simulink library "simetranss"  (R2024b)
settings: Solver=VariableStepAuto  StartTime=0.0  StopTime=10.0  RelTol=1e-3
PostLoadFcn:
  | Ts=1e-6
InitFcn:
  | Ts=1e-6
undefined symbols (not defined in the file): C, C_601, C_603, C_606, CC, Csnu, Csnubber, DiscIntNeverNeededParam, DPL, DPL1ph, FluxTable, ft2km, gcbh, h, Half, Imap2, L, L_601, L_603, L_606, Lbase, LpejoSw, Newton, R_601, R_603, R_606, Raphson, ResistanceM, Roff, Ron, RotorAngles, Rsnu, Rsnubber, Rt4, SampleTime, simetran, sps, sps_rtmsupport, StatorCurrents, T_2wind_ratio, T_Lpu, T_Lpu_pri, T_Rpu, T_Rpu_pri, T_Vpri, T_Vpri_15comp, T_Vsec, Ti, Ts_Power, Z, Zbase, Zm
libraries: fl_lib x248, ee_lib x146, nesl_utility x122, $bdroot x29, simulink x15, eeGeneralControl x2, spsStairGeneratorLib x2, artemis x1
(part 4 of 12)

== system simetranss/FPGA/MATE 2-level inverter backup ==
  gate : Inport
  Demux2 : Demux  Outputs=2
  Pejovic L/C switch2 : Subsystem  mask(Pejovic Switch){Lon=Lon, Ts=Ts}
      mask prompts: Lon "Selected equivalent ON inductance (H)"; Ts "Sample Time (s)"
      mask help:
      | Pevovic switch model in SimScape
      |
      | In the Pejovic model, Ts/Lon=Coff/Ts (Backward Euler)
      |
      |
      | Implements a single phase switch model using the Pejovic constant admittance method.
      | The user only has to select the equivalent ON-state inductance of the model, the corresponding Capacitance is computed internally.
      |
      | Input signals;
      |
      | sw: the switch gate value (1 for ON , 0 for OFF)
      mask init:
      | Coff=Ts*Ts/Lon;
      | Rsw=Lon/Ts;
      | 
      | if Ts>2e-6
      |     warndlg(['Sample Time of ' num2str(Ts) ' s. may be somehow large for the Pejovic switch to be accurate. Sample time below 2 us are recommended.'])
      | end
      mask Display: disp(['Pswitch'])
  Pejovic L/C switch3 : Subsystem  mask(Pejovic Switch){Lon=Lon, Ts=Ts}
      mask prompts: Lon "Selected equivalent ON inductance (H)"; Ts "Sample Time (s)"
      mask help:
      | Pevovic switch model in SimScape
      |
      | In the Pejovic model, Ts/Lon=Coff/Ts (Backward Euler)
      |
      |
      | Implements a single phase switch model using the Pejovic constant admittance method.
      | The user only has to select the equivalent ON-state inductance of the model, the corresponding Capacitance is computed internally.
      |
      | Input signals;
      |
      | sw: the switch gate value (1 for ON , 0 for OFF)
      mask init:
      | Coff=Ts*Ts/Lon;
      | Rsw=Lon/Ts;
      | 
      | if Ts>2e-6
      |     warndlg(['Sample Time of ' num2str(Ts) ' s. may be somehow large for the Pejovic switch to be accurate. Sample time below 2 us are recommended.'])
      | end
      mask Display: disp(['Pswitch'])
  V+ : PMIOPort  Side=Left
  Vout : PMIOPort  Port=2  Side=Right
  V- : PMIOPort  Port=3  Side=Left
  wires:
  Pejovic L/C switch3/2(Xout) -> Pejovic L/C switch2/2(Xin)
  Pejovic L/C switch2/2(Xout) -> Pejovic L/C switch3/2(Xin)
  gate/1 -> Demux2/1
  Demux2/1 -> Pejovic L/C switch2/1(gate)
  Demux2/2 -> Pejovic L/C switch3/1(gate)
  connections:
  Pejovic L/C switch3/RConn1 -- V-/RConn1
  V+/RConn1 -- Pejovic L/C switch2/LConn1
  Pejovic L/C switch3/LConn1 -- Pejovic L/C switch2/RConn1 -- Vout/RConn1

== system simetranss/FPGA/MATE 2level_Inverter SwitchingFunction(2ph) ==
  g : Inport
  Add : Sum  Inputs=+
  Controlled Current Source1 : fl_lib/Electrical/Electrical Sources/Controlled Current Source
  Controlled Voltage Source : fl_lib/Electrical/Electrical Sources/Controlled Voltage Source
  Controlled Voltage Source1 : fl_lib/Electrical/Electrical Sources/Controlled Voltage Source
  Current Sensor : fl_lib/Electrical/Electrical Sensors/Current Sensor
  Current Sensor1 : fl_lib/Electrical/Electrical Sensors/Current Sensor
  Demux : Demux  Outputs=2
  Mux : Mux  Inputs=2
  PS-Simulink Converter : nesl_utility/PS-Simulink Converter  PhysicalDomain=network_engine_domain  SubClassName=ps_output  LeftPortType=input  RightPortType=output  PseudoPeriodic=off  Frequencies=[]  VectorFormat=inherit  Unit=inherit  AffineConversion=off
  PS-Simulink Converter1 : nesl_utility/PS-Simulink Converter  PhysicalDomain=network_engine_domain  SubClassName=ps_output  LeftPortType=input  RightPortType=output  PseudoPeriodic=off  Frequencies=[]  VectorFormat=inherit  Unit=inherit  AffineConversion=off
  PS-Simulink Converter3 : nesl_utility/PS-Simulink Converter  PhysicalDomain=network_engine_domain  SubClassName=ps_output  LeftPortType=input  RightPortType=output  PseudoPeriodic=off  Frequencies=[]  VectorFormat=inherit  Unit=inherit  AffineConversion=off
  Resistor : fl_lib/Electrical/Electrical Elements/Resistor  R=Ron Ohm  i_specify=off  i_priority=None  i=0 A  i_nominal_specify=off  i_nominal_value=1  i_nominal_unit=A  v_specify=off  v_priority=None  v=0 V  v_nominal_specify=off  v_nominal_value=1  v_nominal_unit=V
  Resistor1 : fl_lib/Electrical/Electrical Elements/Resistor  R=Ron Ohm  i_specify=off  i_priority=None  i=0 A  i_nominal_specify=off  i_nominal_value=1  i_nominal_unit=A  v_specify=off  v_priority=None  v=0 V  v_nominal_specify=off  v_nominal_value=1  v_nominal_unit=V
  SW : $bdroot/FPGA/MATE 2level_Inverter  SwitchingFunction(3ph)/SW  SystemSampleTime=-1  VariantActivationTime=update diagram  AllowFlexibleInterface=on  Latency=0  AutoFrameSizeCalculation=off
  Selector : Selector  InputPortWidth=4  IndexOptions=Index vector (dialog)  Indices=[1 3]  OutputSizes=1
  Selector1 : Selector  InputPortWidth=4  IndexOptions=Index vector (dialog)  Indices=[2 4]  OutputSizes=1
  Simulink-PS Converter : nesl_utility/Simulink-PS Converter  PhysicalDomain=network_engine_domain  SubClassName=ps_input  LeftPortType=input  RightPortType=output  PseudoPeriodic=off  Frequencies=[]  NoiseDistribution=none  NoiseParameters=[]  Unit=1  AffineConversion=off  FilteringAndDerivatives=provide  SimscapeFilterOrder=1  InputFilterTimeConstant=0.001  UdotUserProvided=0
  Simulink-PS Converter1 : nesl_utility/Simulink-PS Converter  PhysicalDomain=network_engine_domain  SubClassName=ps_input  LeftPortType=input  RightPortType=output  PseudoPeriodic=off  Frequencies=[]  NoiseDistribution=none  NoiseParameters=[]  Unit=1  AffineConversion=off  FilteringAndDerivatives=provide  SimscapeFilterOrder=1  InputFilterTimeConstant=0.001  UdotUserProvided=0
  Simulink-PS Converter2 : nesl_utility/Simulink-PS Converter  PhysicalDomain=network_engine_domain  SubClassName=ps_input  LeftPortType=input  RightPortType=output  PseudoPeriodic=off  Frequencies=[]  NoiseDistribution=none  NoiseParameters=[]  Unit=1  AffineConversion=off  FilteringAndDerivatives=provide  SimscapeFilterOrder=1  InputFilterTimeConstant=0.001  UdotUserProvided=0
  Unit Delay : UnitDelay  SampleTime=Ts  HasFrameUpgradeWarning=on
  Unit Delay1 : UnitDelay  SampleTime=Ts  HasFrameUpgradeWarning=on
  Voltage Sensor : fl_lib/Electrical/Electrical Sensors/Voltage Sensor
  V+ : PMIOPort  Side=Right
  V- : PMIOPort  Port=2  Side=Right
  + : PMIOPort  Port=3  Side=Left
  - : PMIOPort  Port=4  Side=Left
  wires:
  Add/1 -> Simulink-PS Converter/1
  g/1 -> Selector1/1, Selector/1
  SW/2 -> Unit Delay1/1
  SW/1 -> Unit Delay/1
  Unit Delay/1 -> Add/1
  PS-Simulink Converter1/1 -> SW/3
  PS-Simulink Converter/1 -> Mux/1
  PS-Simulink Converter3/1 -> Mux/2
  Mux/1 -> SW/4
  Demux/2 -> Simulink-PS Converter2/1
  Demux/1 -> Simulink-PS Converter1/1
  Unit Delay1/1 -> Demux/1
  Selector/1 -> SW/1
  Selector1/1 -> SW/2
  connections:
  Current Sensor/RConn2 -- Resistor/LConn1
  Controlled Voltage Source/LConn1 -- Current Sensor/LConn1
  Simulink-PS Converter/RConn1 -- Controlled Current Source1/RConn1
  PS-Simulink Converter/LConn1 -- Current Sensor/RConn1
  Simulink-PS Converter1/RConn1 -- Controlled Voltage Source/RConn1
  Controlled Voltage Source/RConn2 -- Controlled Current Source1/LConn1 -- Voltage Sensor/RConn2 -- V-/RConn1 -- Controlled Voltage Source1/RConn2
  Controlled Current Source1/RConn2 -- Voltage Sensor/LConn1 -- V+/RConn1
  PS-Simulink Converter1/LConn1 -- Voltage Sensor/RConn1
  Current Sensor1/RConn2 -- Resistor1/LConn1
  +/RConn1 -- Resistor/RConn1
  -/RConn1 -- Resistor1/RConn1
  PS-Simulink Converter3/LConn1 -- Current Sensor1/RConn1
  Current Sensor1/LConn1 -- Controlled Voltage Source1/LConn1
  Simulink-PS Converter2/RConn1 -- Controlled Voltage Source1/RConn1

== system simetranss/FPGA/MATE 2level_Inverter SwitchingFunction(3ph) ==
  g : Inport
  Add : Sum  Inputs=+
  Controlled Current Source1 : fl_lib/Electrical/Electrical Sources/Controlled Current Source
  Controlled Voltage Source : fl_lib/Electrical/Electrical Sources/Controlled Voltage Source
  Controlled Voltage Source1 : fl_lib/Electrical/Electrical Sources/Controlled Voltage Source
  Controlled Voltage Source2 : fl_lib/Electrical/Electrical Sources/Controlled Voltage Source
  Current Sensor : fl_lib/Electrical/Electrical Sensors/Current Sensor
  Current Sensor1 : fl_lib/Electrical/Electrical Sensors/Current Sensor
  Current Sensor2 : fl_lib/Electrical/Electrical Sensors/Current Sensor
  Demux : Demux  Outputs=3
  Mux : Mux  Inputs=3
  PS-Simulink Converter{,1..3} (4 alike) : nesl_utility/PS-Simulink Converter  PhysicalDomain=network_engine_domain  SubClassName=ps_output  LeftPortType=input  RightPortType=output  PseudoPeriodic=off  Frequencies=[]  VectorFormat=inherit  Unit=inherit  AffineConversion=off
  Phase Splitter : ee_lib/Connectors & References/Phase Splitter
  Resistor : fl_lib/Electrical/Electrical Elements/Resistor  R=Ron Ohm  i_specify=off  i_priority=None  i=0 A  i_nominal_specify=off  i_nominal_value=1  i_nominal_unit=A  v_specify=off  v_priority=None  v=0 V  v_nominal_specify=off  v_nominal_value=1  v_nominal_unit=V
  Resistor1 : fl_lib/Electrical/Electrical Elements/Resistor  R=Ron Ohm  i_specify=off  i_priority=None  i=0 A  i_nominal_specify=off  i_nominal_value=1  i_nominal_unit=A  v_specify=off  v_priority=None  v=0 V  v_nominal_specify=off  v_nominal_value=1  v_nominal_unit=V
  Resistor2 : fl_lib/Electrical/Electrical Elements/Resistor  R=Ron Ohm  i_specify=off  i_priority=None  i=0 A  i_nominal_specify=off  i_nominal_value=1  i_nominal_unit=A  v_specify=off  v_priority=None  v=0 V  v_nominal_specify=off  v_nominal_value=1  v_nominal_unit=V
  SW : Subsystem
  Selector : Selector  InputPortWidth=6  IndexOptions=Index vector (dialog)  Indices=[1 3 5]  OutputSizes=1
  Selector1 : Selector  InputPortWidth=6  IndexOptions=Index vector (dialog)  Indices=[1 3 5]+1  OutputSizes=1
  Simulink-PS Converter{,1..3} (4 alike) : nesl_utility/Simulink-PS Converter  PhysicalDomain=network_engine_domain  SubClassName=ps_input  LeftPortType=input  RightPortType=output  PseudoPeriodic=off  Frequencies=[]  NoiseDistribution=none  NoiseParameters=[]  Unit=1  AffineConversion=off  FilteringAndDerivatives=provide  SimscapeFilterOrder=1  InputFilterTimeConstant=0.001  UdotUserProvided=0
  Unit Delay : UnitDelay  SampleTime=Ts  HasFrameUpgradeWarning=on
  Unit Delay1 : UnitDelay  SampleTime=Ts  HasFrameUpgradeWarning=on
  Voltage Sensor : fl_lib/Electrical/Electrical Sensors/Voltage Sensor
  abc : PMIOPort  Side=Left
  V+ : PMIOPort  Port=2  Side=Right
  V- : PMIOPort  Port=3  Side=Right
  wires:
  Selector1/1 -> SW/2(gl)
  Selector/1 -> SW/1(gu)
  Unit Delay1/1 -> Demux/1
  Demux/1 -> Simulink-PS Converter1/1
  Demux/2 -> Simulink-PS Converter2/1
  Demux/3 -> Simulink-PS Converter3/1
  Mux/1 -> SW/4(Iac)
  PS-Simulink Converter2/1 -> Mux/3
  PS-Simulink Converter3/1 -> Mux/2
  PS-Simulink Converter/1 -> Mux/1
  PS-Simulink Converter1/1 -> SW/3(Vdc)
  Unit Delay/1 -> Add/1
  SW/1(Idc) -> Unit Delay/1
  SW/2(Vac) -> Unit Delay1/1
  g/1 -> Selector/1, Selector1/1
  Add/1 -> Simulink-PS Converter/1
  connections:
  Controlled Voltage Source2/LConn1 -- Current Sensor2/LConn1
  Simulink-PS Converter3/RConn1 -- Controlled Voltage Source2/RConn1
  Simulink-PS Converter2/RConn1 -- Controlled Voltage Source1/RConn1
  Current Sensor1/LConn1 -- Controlled Voltage Source1/LConn1
  PS-Simulink Converter2/LConn1 -- Current Sensor2/RConn1
  PS-Simulink Converter3/LConn1 -- Current Sensor1/RConn1
  Resistor2/RConn1 -- Phase Splitter/RConn3
  Resistor1/RConn1 -- Phase Splitter/RConn2
  Resistor/RConn1 -- Phase Splitter/RConn1
  Phase Splitter/LConn1 -- abc/RConn1
  Current Sensor2/RConn2 -- Resistor2/LConn1
  Current Sensor1/RConn2 -- Resistor1/LConn1
  PS-Simulink Converter1/LConn1 -- Voltage Sensor/RConn1
  V+/RConn1 -- Voltage Sensor/LConn1 -- Controlled Current Source1/RConn2
  Controlled Voltage Source2/RConn2 -- Controlled Voltage Source1/RConn2 -- V-/RConn1 -- Voltage Sensor/RConn2 -- Controlled Current Source1/LConn1 -- Controlled Voltage Source/RConn2
  Simulink-PS Converter1/RConn1 -- Controlled Voltage Source/RConn1
  PS-Simulink Converter/LConn1 -- Current Sensor/RConn1
  Simulink-PS Converter/RConn1 -- Controlled Current Source1/RConn1
  Controlled Voltage Source/LConn1 -- Current Sensor/LConn1
  Current Sensor/RConn2 -- Resistor/LConn1

== system simetranss/FPGA/MATE 2level_InverterSWHIZ ==
  g : Inport
  CCS : fl_lib/Electrical/Electrical Sources/Controlled Current Source
  CVS : fl_lib/Electrical/Electrical Sources/Controlled Voltage Source
  Constant : Constant  Value=[Gpp Ts/Gip min_charge]
  Isensor : fl_lib/Electrical/Electrical Sensors/Current Sensor
  PS-Simulink Converter : nesl_utility/PS-Simulink Converter  PhysicalDomain=network_engine_domain  SubClassName=ps_output  LeftPortType=input  RightPortType=output  PseudoPeriodic=off  Frequencies=[]  VectorFormat=inherit  Unit=inherit  AffineConversion=off
  PS-Simulink Converter1 : nesl_utility/PS-Simulink Converter  PhysicalDomain=network_engine_domain  SubClassName=ps_output  LeftPortType=input  RightPortType=output  PseudoPeriodic=off  Frequencies=[]  VectorFormat=inherit  Unit=inherit  AffineConversion=off
  R : fl_lib/Electrical/Electrical Elements/Resistor  R=Ron Ohm  i_specify=off  i_priority=None  i=0 A  i_nominal_specify=off  i_nominal_value=1  i_nominal_unit=A  v_specify=off  v_priority=None  v=0 V  v_nominal_specify=off  v_nominal_value=1  v_nominal_unit=V
  SW : Subsystem
  Selector : Selector  InputPortWidth=2  IndexOptions=Index vector (dialog)  Indices=[1 ]  OutputSizes=1
  Selector1 : Selector  InputPortWidth=2  IndexOptions=Index vector (dialog)  Indices=[2 ]  OutputSizes=1
  Simulink-PS Converter : nesl_utility/Simulink-PS Converter  PhysicalDomain=network_engine_domain  SubClassName=ps_input  LeftPortType=input  RightPortType=output  PseudoPeriodic=off  Frequencies=[]  NoiseDistribution=none  NoiseParameters=[]  Unit=1  AffineConversion=off  FilteringAndDerivatives=provide  SimscapeFilterOrder=1  InputFilterTimeConstant=0.001  UdotUserProvided=0
  Simulink-PS Converter1 : nesl_utility/Simulink-PS Converter  PhysicalDomain=network_engine_domain  SubClassName=ps_input  LeftPortType=input  RightPortType=output  PseudoPeriodic=off  Frequencies=[]  NoiseDistribution=none  NoiseParameters=[]  Unit=1  AffineConversion=off  FilteringAndDerivatives=provide  SimscapeFilterOrder=1  InputFilterTimeConstant=0.001  UdotUserProvided=0
  Unit Delay2 : UnitDelay  SampleTime=Ts  HasFrameUpgradeWarning=on
  Unit Delay3 : UnitDelay  SampleTime=Ts  HasFrameUpgradeWarning=on
  Vsensor : fl_lib/Electrical/Electrical Sensors/Voltage Sensor
  V+ : PMIOPort  Side=Left
  V- : PMIOPort  Port=2  Side=Left
  A : PMIOPort  Port=3  Side=Right
  wires:
  Constant/1 -> SW/5(params)
  Unit Delay3/1 -> SW/3(Vdc)
  Unit Delay2/1 -> SW/4(Iac)
  SW/2(Vac) -> Simulink-PS Converter1/1
  SW/1(Idc) -> Simulink-PS Converter/1
  g/1 -> Selector/1, Selector1/1
  PS-Simulink Converter1/1 -> Unit Delay3/1
  PS-Simulink Converter/1 -> Unit Delay2/1
  Selector/1 -> SW/1(gu)
  Selector1/1 -> SW/2(gl)
  connections:
  Isensor/RConn2 -- CVS/LConn1
  R/LConn1 -- Isensor/LConn1
  Simulink-PS Converter/RConn1 -- CCS/RConn1
  PS-Simulink Converter/LConn1 -- Isensor/RConn1
  Simulink-PS Converter1/RConn1 -- CVS/RConn1
  CCS/LConn1 -- Vsensor/RConn2 -- V-/RConn1 -- CVS/RConn2
  CCS/RConn2 -- Vsensor/LConn1 -- V+/RConn1
  PS-Simulink Converter1/LConn1 -- Vsensor/RConn1
  A/RConn1 -- R/RConn1

== system simetranss/FPGA/MATE 3levelNPC_Inverter SwitchingFunction(3ph) ==
  g : Inport
  Add : Sum  Inputs=+
  Add1 : Sum  Inputs=+
  Controlled Current Source1 : fl_lib/Electrical/Electrical Sources/Controlled Current Source
  Controlled Current Source2 : fl_lib/Electrical/Electrical Sources/Controlled Current Source
  Controlled Voltage Source : fl_lib/Electrical/Electrical Sources/Controlled Voltage Source
  Controlled Voltage Source1 : fl_lib/Electrical/Electrical Sources/Controlled Voltage Source
  Controlled Voltage Source2 : fl_lib/Electrical/Electrical Sources/Controlled Voltage Source
  Current Sensor : fl_lib/Electrical/Electrical Sensors/Current Sensor
  Current Sensor1 : fl_lib/Electrical/Electrical Sensors/Current Sensor
  Current Sensor2 : fl_lib/Electrical/Electrical Sensors/Current Sensor
  Demux : Demux  Outputs=3
  Mux : Mux  Inputs=3
  PS-Simulink Converter{,1..4} (5 alike) : nesl_utility/PS-Simulink Converter  PhysicalDomain=network_engine_domain  SubClassName=ps_output  LeftPortType=input  RightPortType=output  PseudoPeriodic=off  Frequencies=[]  VectorFormat=inherit  Unit=inherit  AffineConversion=off
  Phase Splitter : ee_lib/Connectors & References/Phase Splitter
  Q1 : Selector  InputPortWidth=12  IndexOptions=Index vector (dialog)  Indices=[1 5 9]  OutputSizes=[(-2)]
  Q2 : Selector  InputPortWidth=12  IndexOptions=Index vector (dialog)  Indices=[1 5 9]+1  OutputSizes=[(-2)]
  Q3 : Selector  InputPortWidth=12  IndexOptions=Index vector (dialog)  Indices=[1 5 9]+2  OutputSizes=[(-2)]
  Q4 : Selector  InputPortWidth=12  IndexOptions=Index vector (dialog)  Indices=[1 5 9]+3  OutputSizes=[(-2)]
  Resistor : fl_lib/Electrical/Electrical Elements/Resistor  R=2*Ron Ohm  i_specify=off  i_priority=None  i=0 A  i_nominal_specify=off  i_nominal_value=1  i_nominal_unit=A  v_specify=off  v_priority=None  v=0 V  v_nominal_specify=off  v_nominal_value=1  v_nominal_unit=V
  Resistor1 : fl_lib/Electrical/Electrical Elements/Resistor  R=2*Ron Ohm  i_specify=off  i_priority=None  i=0 A  i_nominal_specify=off  i_nominal_value=1  i_nominal_unit=A  v_specify=off  v_priority=None  v=0 V  v_nominal_specify=off  v_nominal_value=1  v_nominal_unit=V
  Resistor2 : fl_lib/Electrical/Electrical Elements/Resistor  R=2*Ron Ohm  i_specify=off  i_priority=None  i=0 A  i_nominal_specify=off  i_nominal_value=1  i_nominal_unit=A  v_specify=off  v_priority=None  v=0 V  v_nominal_specify=off  v_nominal_value=1  v_nominal_unit=V
  SW : Subsystem
  Simulink-PS Converter{,1..4} (5 alike) : nesl_utility/Simulink-PS Converter  PhysicalDomain=network_engine_domain  SubClassName=ps_input  LeftPortType=input  RightPortType=output  PseudoPeriodic=off  Frequencies=[]  NoiseDistribution=none  NoiseParameters=[]  Unit=1  AffineConversion=off  FilteringAndDerivatives=provide  SimscapeFilterOrder=1  InputFilterTimeConstant=0.001  UdotUserProvided=0
  Unit Delay : UnitDelay  SampleTime=Ts  HasFrameUpgradeWarning=on
  Unit Delay1 : UnitDelay  SampleTime=Ts  HasFrameUpgradeWarning=on
  Unit Delay2 : UnitDelay  SampleTime=Ts  HasFrameUpgradeWarning=on
  Voltage Sensor : fl_lib/Electrical/Electrical Sensors/Voltage Sensor
  Voltage Sensor1 : fl_lib/Electrical/Electrical Sensors/Voltage Sensor
  abc : PMIOPort  Side=Right
  V+ : PMIOPort  Port=2  Side=Left
  Vn : PMIOPort  Port=3  Side=Left
  V- : PMIOPort  Port=4  Side=Left
  wires:
  Q4/1 -> SW/4(g4)
  Q3/1 -> SW/3(g3)
  Q2/1 -> SW/2(g2)
  Q1/1 -> SW/1(g1)
  Unit Delay1/1 -> Demux/1
  Demux/1 -> Simulink-PS Converter1/1
  Demux/2 -> Simulink-PS Converter2/1
  Demux/3 -> Simulink-PS Converter3/1
  Mux/1 -> SW/6(Iac)
  PS-Simulink Converter2/1 -> Mux/3
  PS-Simulink Converter3/1 -> Mux/2
  PS-Simulink Converter/1 -> Mux/1
  PS-Simulink Converter1/1 -> SW/5(VPM)
  Unit Delay/1 -> Add/1
  SW/1(IdcPM) -> Unit Delay/1
  SW/3(Vac) -> Unit Delay1/1
  Add/1 -> Simulink-PS Converter/1
  PS-Simulink Converter4/1 -> SW/7(VNM)
  Add1/1 -> Simulink-PS Converter4/1
  Unit Delay2/1 -> Add1/1
  SW/2(IdcNM) -> Unit Delay2/1
  g/1 -> Q2/1, Q3/1, Q4/1, Q1/1
  connections:
  Controlled Voltage Source2/LConn1 -- Current Sensor2/LConn1
  Simulink-PS Converter3/RConn1 -- Controlled Voltage Source2/RConn1
  Simulink-PS Converter2/RConn1 -- Controlled Voltage Source1/RConn1
  Current Sensor1/LConn1 -- Controlled Voltage Source1/LConn1
  PS-Simulink Converter2/LConn1 -- Current Sensor2/RConn1
  PS-Simulink Converter3/LConn1 -- Current Sensor1/RConn1
  Resistor2/RConn1 -- Phase Splitter/RConn3
  Resistor1/RConn1 -- Phase Splitter/RConn2
  Resistor/RConn1 -- Phase Splitter/RConn1
  Phase Splitter/LConn1 -- abc/RConn1
  Current Sensor2/RConn2 -- Resistor2/LConn1
  Current Sensor1/RConn2 -- Resistor1/LConn1
  PS-Simulink Converter1/LConn1 -- Voltage Sensor/RConn1
  V+/RConn1 -- Voltage Sensor/LConn1 -- Controlled Current Source1/RConn2
  V-/RConn1 -- Voltage Sensor1/RConn2 -- Voltage Sensor/RConn2 -- Controlled Voltage Source2/RConn2 -- Controlled Voltage Source1/RConn2 -- Controlled Voltage Source/RConn2 -- Controlled Current Source1/LConn1 -- Controlled Current Source2/LConn1
  Simulink-PS Converter1/RConn1 -- Controlled Voltage Source/RConn1
  PS-Simulink Converter/LConn1 -- Current Sensor/RConn1
  Simulink-PS Converter/RConn1 -- Controlled Current Source1/RConn1
  Controlled Voltage Source/LConn1 -- Current Sensor/LConn1
  Current Sensor/RConn2 -- Resistor/LConn1
  Voltage Sensor1/LConn1 -- Vn/RConn1 -- Controlled Current Source2/RConn2
  Voltage Sensor1/RConn1 -- PS-Simulink Converter4/LConn1
  Simulink-PS Converter4/RConn1 -- Controlled Current Source2/RConn1

== system simetranss/FPGA/Pejovic L-C-switch component ==
  Add : Sum  Inputs=+-
  CCS1 : fl_lib/Electrical/Electrical Sources/Controlled Current Source
  Gain1 : Gain  Gain=-1/Rsw
  Gain2 : Gain  Gain=Xcomp
  Gain3 : Gain  Gain=-1
  PS-Simulink Converter2 : nesl_utility/PS-Simulink Converter  PhysicalDomain=network_engine_domain  SubClassName=ps_output  LeftPortType=input  RightPortType=output  PseudoPeriodic=off  Frequencies=[]  VectorFormat=inherit  Unit=inherit  AffineConversion=off
  Relational Operator1 : RelationalOperator  Operator=~=  OutDataTypeStr=boolean  RndMeth=Simplest  InputSameDT=off
  Resistor : fl_lib/Electrical/Electrical Elements/Resistor  R=Rsw Ohm  i_specify=off  i_priority=None  i=0 A  i_nominal_specify=off  i_nominal_value=1  i_nominal_unit=A  v_specify=off  v_priority=None  v=0 V  v_nominal_specify=off  v_nominal_value=1  v_nominal_unit=V
  Simulink-PS Converter1 : nesl_utility/Simulink-PS Converter  PhysicalDomain=network_engine_domain  SubClassName=ps_input  LeftPortType=input  RightPortType=output  PseudoPeriodic=off  Frequencies=[]  NoiseDistribution=none  NoiseParameters=[]  Unit=1  AffineConversion=off  FilteringAndDerivatives=provide  SimscapeFilterOrder=1  InputFilterTimeConstant=0.001  UdotUserProvided=0
  Switch : Switch  Criteria=u2 > Threshold  Threshold=0.5  SaturateOnIntegerOverflow=off  InputSameDT=off
  Switch4 : Switch  Criteria=u2 > Threshold  Threshold=0.5  SaturateOnIntegerOverflow=off  InputSameDT=off
  Switch5 : Switch  Criteria=u2 > Threshold  Threshold=0.5  SaturateOnIntegerOverflow=off  InputSameDT=off
  Unit Delay1 : UnitDelay  SampleTime=-1  HasFrameUpgradeWarning=on
  Unit Delay5 : UnitDelay  SampleTime=Ts  HasFrameUpgradeWarning=on
  Unit Delay6 : UnitDelay  SampleTime=Ts  HasFrameUpgradeWarning=on
  VS1 : fl_lib/Electrical/Electrical Sensors/Voltage Sensor
  gate : Constant
  init_in : Constant
  init_out : Terminator
  +V : PMIOPort  Side=Left
  -V : PMIOPort  Port=2  Side=Right
  wires:
  Switch5/1 -> [Ihist]
  init_in/1 -> Switch5/1
  Relational Operator1/1 -> Gain2/1
  gate/1 -> Switch/2, Relational Operator1/2, Unit Delay6/1, Switch4/2
  Unit Delay6/1 -> Relational Operator1/1
  Gain2/1 -> Switch5/2
  Gain3/1 -> Switch4/1
  Switch4/1 -> Unit Delay5/1
  [Isw] -> Gain3/1
  Unit Delay5/1 -> init_out/1
  Unit Delay1/1 -> Switch5/3
  Add/1 -> Switch/1, [Isw]
  Gain1/1 -> Add/2, Switch/3, Switch4/3
  [Ihist] -> Add/1
  PS-Simulink Converter2/1 -> [Vsw]
  [Vsw] -> Gain1/1
  Switch/1 -> Unit Delay1/1
  [Ihist] -> Simulink-PS Converter1/1
  connections:
  Resistor/RConn1 -- CCS1/LConn1 -- VS1/RConn2 -- -V/RConn1
  PS-Simulink Converter2/LConn1 -- VS1/RConn1
  CCS1/RConn1 -- Simulink-PS Converter1/RConn1
  Resistor/LConn1 -- VS1/LConn1 -- +V/RConn1 -- CCS1/RConn2

== system simetranss/FPGA/Pejovic L//C switch ==
  gate : Inport
  Bus Creator : BusCreator  Inputs=2
  Controlled Current Source : fl_lib/Electrical/Electrical Sources/Controlled Current Source
  Current Sensor : fl_lib/Electrical/Electrical Sensors/Current Sensor
  Gain : Gain  Gain=-1
  Gain1 : Gain  Gain=1/Rsw
  PS-Simulink Converter1 : nesl_utility/PS-Simulink Converter  PhysicalDomain=network_engine_domain  SubClassName=ps_output  LeftPortType=input  RightPortType=output  PseudoPeriodic=off  Frequencies=[]  VectorFormat=inherit  Unit=inherit  AffineConversion=off
  PS-Simulink Converter2 : nesl_utility/PS-Simulink Converter  PhysicalDomain=network_engine_domain  SubClassName=ps_output  LeftPortType=input  RightPortType=output  PseudoPeriodic=off  Frequencies=[]  VectorFormat=inherit  Unit=inherit  AffineConversion=off
  Resistor : fl_lib/Electrical/Electrical Elements/Resistor  R=Rsw Ohm  i_specify=off  i_priority=None  i=0 A  i_nominal_specify=off  i_nominal_value=1  i_nominal_unit=A  v_specify=off  v_priority=None  v=0 V  v_nominal_specify=off  v_nominal_value=1  v_nominal_unit=V
  Simulink-PS Converter1 : nesl_utility/Simulink-PS Converter  PhysicalDomain=network_engine_domain  SubClassName=ps_input  LeftPortType=input  RightPortType=output  PseudoPeriodic=off  Frequencies=[]  NoiseDistribution=none  NoiseParameters=[]  Unit=1  AffineConversion=off  FilteringAndDerivatives=provide  SimscapeFilterOrder=1  InputFilterTimeConstant=0.001  UdotUserProvided=0
  Switch : Switch  Criteria=u2 > Threshold  Threshold=0.5  SaturateOnIntegerOverflow=off  InputSameDT=off
  Unit Delay : UnitDelay  SampleTime=-1  HasFrameUpgradeWarning=on
  Voltage Sensor : fl_lib/Electrical/Electrical Sensors/Voltage Sensor
  +V : PMIOPort  Side=Left
  -V : PMIOPort  Port=2  Side=Right
  meas : Outport
  wires:
  PS-Simulink Converter2/1 -> [Vsw]
  PS-Simulink Converter1/1 -> [Isw]
  gate/1 -> Switch/2
  Switch/1 -> Unit Delay/1
  [Isw] -> Gain/1
  Gain/1 -> Switch/1
  [Vsw] -> Gain1/1
  Gain1/1 -> Switch/3
  Unit Delay/1 -> [Ihist]
  [Ihist] -> Simulink-PS Converter1/1
  [Isw] -> Bus Creator/2  "Switch current (A)"
  [Vsw] -> Bus Creator/1  "Switch voltage (V)"
  Bus Creator/1 -> meas/1
  connections:
  Resistor/RConn1 -- Voltage Sensor/RConn2 -- -V/RConn1 -- Controlled Current Source/RConn2
  Current Sensor/RConn2 -- Voltage Sensor/LConn1 -- Resistor/LConn1 -- Controlled Current Source/LConn1
  PS-Simulink Converter2/LConn1 -- Voltage Sensor/RConn1
  Controlled Current Source/RConn1 -- Simulink-PS Converter1/RConn1
  +V/RConn1 -- Current Sensor/LConn1
  Current Sensor/RConn1 -- PS-Simulink Converter1/LConn1

== system simetranss/Lines/Half-DPL ==
  Zvi_in : Inport
  Demux : Demux  Outputs=3
      settings: DisplayOption=none
  Electrical Reference1 : fl_lib/Electrical/Electrical Elements/Electrical Reference
  Electrical Reference2 : fl_lib/Electrical/Electrical Elements/Electrical Reference
  Electrical Reference3 : fl_lib/Electrical/Electrical Elements/Electrical Reference
  Mux : Mux  Inputs=3
  Phase Splitter1 : ee_lib/Connectors & References/Phase Splitter
  Resistor1 : ee_lib/Passive/Resistor  R=ResistanceM(1,1) Ohm  enable_R_tol=ee.enum.toleranceApplication.none  R_tol=5  tol_distribution=ee.enum.toleranceDistribution.uniform  nSigma=4  enable_operating_limits=ee.enum.enable.no  operating_limit_action=ee.enum.passive.reportOpLim.warn  power_rating=1 W  max_working_voltage=100 V  noise_mode=ee.enum.sources.noise.Disabled  Tdevice=25 degC  sample_time=1e-3 s  repeatability=ee.enum.ic.repeatability.notRepeatable  user_seed=0  auto_seed=3886434167  fault_action=simscape.enum.assert.action.none  t_fault=1 s  power_derating_T1=70 degC  power_derating_T2=155 degC  operating_temperature_range_vec=[-50, 150] degC  alpha=3.93e-3 1/K  Tmeas=25 degC  thermal_mass=100 J/K  temperature_specify=off  temperature_priority=High  temperature=298.15 K  temperature_nominal_specify=off  temperature_nominal_value=1  temperature_nominal_unit=K
  Resistor2 : ee_lib/Passive/Resistor  R=ResistanceM(2,2) Ohm  enable_R_tol=ee.enum.toleranceApplication.none  R_tol=5  tol_distribution=ee.enum.toleranceDistribution.uniform  nSigma=4  enable_operating_limits=ee.enum.enable.no  operating_limit_action=ee.enum.passive.reportOpLim.warn  power_rating=1 W  max_working_voltage=100 V  noise_mode=ee.enum.sources.noise.Disabled  Tdevice=25 degC  sample_time=1e-3 s  repeatability=ee.enum.ic.repeatability.notRepeatable  user_seed=0  auto_seed=4207987243  fault_action=simscape.enum.assert.action.none  t_fault=1 s  power_derating_T1=70 degC  power_derating_T2=155 degC  operating_temperature_range_vec=[-50, 150] degC  alpha=3.93e-3 1/K  Tmeas=25 degC  thermal_mass=100 J/K  temperature_specify=off  temperature_priority=High  temperature=298.15 K  temperature_nominal_specify=off  temperature_nominal_value=1  temperature_nominal_unit=K
  Resistor3 : ee_lib/Passive/Resistor  R=ResistanceM(3,3) Ohm  enable_R_tol=ee.enum.toleranceApplication.none  R_tol=5  tol_distribution=ee.enum.toleranceDistribution.uniform  nSigma=4  enable_operating_limits=ee.enum.enable.no  operating_limit_action=ee.enum.passive.reportOpLim.warn  power_rating=1 W  max_working_voltage=100 V  noise_mode=ee.enum.sources.noise.Disabled  Tdevice=25 degC  sample_time=1e-3 s  repeatability=ee.enum.ic.repeatability.notRepeatable  user_seed=0  auto_seed=1884932182  fault_action=simscape.enum.assert.action.none  t_fault=1 s  power_derating_T1=70 degC  power_derating_T2=155 degC  operating_temperature_range_vec=[-50, 150] degC  alpha=3.93e-3 1/K  Tmeas=25 degC  thermal_mass=100 J/K  temperature_specify=off  temperature_priority=High  temperature=298.15 K  temperature_nominal_specify=off  temperature_nominal_value=1  temperature_nominal_unit=K
  Resistor4 : ee_lib/Passive/Resistor  R=ResistanceM(1,2) Ohm  enable_R_tol=ee.enum.toleranceApplication.none  R_tol=5  tol_distribution=ee.enum.toleranceDistribution.uniform  nSigma=4  enable_operating_limits=ee.enum.enable.no  operating_limit_action=ee.enum.passive.reportOpLim.warn  power_rating=1 W  max_working_voltage=100 V  noise_mode=ee.enum.sources.noise.Disabled  Tdevice=25 degC  sample_time=1e-3 s  repeatability=ee.enum.ic.repeatability.notRepeatable  user_seed=0  auto_seed=477253431  fault_action=simscape.enum.assert.action.none  t_fault=1 s  power_derating_T1=70 degC  power_derating_T2=155 degC  operating_temperature_range_vec=[-50, 150] degC  alpha=3.93e-3 1/K  Tmeas=25 degC  thermal_mass=100 J/K  temperature_specify=off  temperature_priority=High  temperature=298.15 K  temperature_nominal_specify=off  temperature_nominal_value=1  temperature_nominal_unit=K
  Resistor5 : ee_lib/Passive/Resistor  R=ResistanceM(2,3) Ohm  enable_R_tol=ee.enum.toleranceApplication.none  R_tol=5  tol_distribution=ee.enum.toleranceDistribution.uniform  nSigma=4  enable_operating_limits=ee.enum.enable.no  operating_limit_action=ee.enum.passive.reportOpLim.warn  power_rating=1 W  max_working_voltage=100 V  noise_mode=ee.enum.sources.noise.Disabled  Tdevice=25 degC  sample_time=1e-3 s  repeatability=ee.enum.ic.repeatability.notRepeatable  user_seed=0  auto_seed=1108379429  fault_action=simscape.enum.assert.action.none  t_fault=1 s  power_derating_T1=70 degC  power_derating_T2=155 degC  operating_temperature_range_vec=[-50, 150] degC  alpha=3.93e-3 1/K  Tmeas=25 degC  thermal_mass=100 J/K  temperature_specify=off  temperature_priority=High  temperature=298.15 K  temperature_nominal_specify=off  temperature_nominal_value=1  temperature_nominal_unit=K
  Resistor6 : ee_lib/Passive/Resistor  R=ResistanceM(1,3) Ohm  enable_R_tol=ee.enum.toleranceApplication.none  R_tol=5  tol_distribution=ee.enum.toleranceDistribution.uniform  nSigma=4  enable_operating_limits=ee.enum.enable.no  operating_limit_action=ee.enum.passive.reportOpLim.warn  power_rating=1 W  max_working_voltage=100 V  noise_mode=ee.enum.sources.noise.Disabled  Tdevice=25 degC  sample_time=1e-3 s  repeatability=ee.enum.ic.repeatability.notRepeatable  user_seed=0  auto_seed=1755438372  fault_action=simscape.enum.assert.action.none  t_fault=1 s  power_derating_T1=70 degC  power_derating_T2=155 degC  operating_temperature_range_vec=[-50, 150] degC  alpha=3.93e-3 1/K  Tmeas=25 degC  thermal_mass=100 J/K  temperature_specify=off  temperature_priority=High  temperature=298.15 K  temperature_nominal_specify=off  temperature_nominal_value=1  temperature_nominal_unit=K
  Simscape : Subsystem
      mask Display: disp('V')
  Simscape1 : Subsystem
      mask Display: disp('V')
  Simscape2 : Subsystem
      mask Display: disp('V')
  Voltage Source : Subsystem
  Voltage Source1 : Subsystem
  Voltage Source2 : Subsystem
  dplmodel : Subsystem
  gnd : fl_lib/Electrical/Electrical Elements/Electrical Reference
  gnd1 : fl_lib/Electrical/Electrical Elements/Electrical Reference
  gnd2 : fl_lib/Electrical/Electrical Elements/Electrical Reference
  abc : PMIOPort  Side=Left
  Zvi_out : Outport  VectorParamsAs1DForOutWhenUnconnected=off
  Vnode : Outport  Port=2  VectorParamsAs1DForOutWhenUnconnected=off
  wires:
  [I_A_1] -> Voltage Source/1(I)
  Simscape1/1(Out) -> [V_A_2]
  Simscape/1(Out) -> [V_A_1]
  [I_A_3] -> Voltage Source2/1(I)
  Simscape2/1(Out) -> [V_A_3]
  [I_A_2] -> Voltage Source1/1(I)
  dplmodel/2(hist_out) -> [ho]
  [hi] -> dplmodel/2(hist_in)
  Zvi_in/1 -> [hi]
  Mux/1 -> dplmodel/1(v), Vnode/1
  dplmodel/1(i) -> Demux/1
  [V_A_1] -> Mux/1
  Demux/1 -> [I_A_1]
  [V_A_2] -> Mux/2
  Demux/2 -> [I_A_2]
  [V_A_3] -> Mux/3
  Demux/3 -> [I_A_3]
  [ho] -> Zvi_out/1
  connections:
  abc/RConn1 -- Phase Splitter1/LConn1
  Resistor3/LConn1 -- gnd2/LConn1
  Electrical Reference1/LConn1 -- Voltage Source/RConn2
  Resistor2/LConn1 -- gnd1/LConn1
  Resistor1/LConn1 -- gnd/LConn1
  Electrical Reference3/LConn1 -- Voltage Source2/RConn2
  Electrical Reference2/LConn1 -- Voltage Source1/RConn2
  Phase Splitter1/RConn2 -- Resistor4/RConn1 -- Simscape1/LConn1 -- Voltage Source1/RConn1 -- Resistor2/RConn1 -- Resistor5/LConn1
  Phase Splitter1/RConn3 -- Resistor3/RConn1 -- Voltage Source2/RConn1 -- Simscape2/LConn1 -- Resistor5/RConn1 -- Resistor6/RConn1
  Phase Splitter1/RConn1 -- Resistor6/LConn1 -- Resistor4/LConn1 -- Resistor1/RConn1 -- Voltage Source/RConn1 -- Simscape/LConn1

== system simetranss/Lines/Half-DPL1ph ==
  Zvi_in : Inport
  Electrical Reference1 : fl_lib/Electrical/Electrical Elements/Electrical Reference
  Resistor1 : ee_lib/Passive/Resistor  R=ResistanceM(1,1) Ohm  enable_R_tol=ee.enum.toleranceApplication.none  R_tol=5  tol_distribution=ee.enum.toleranceDistribution.uniform  nSigma=4  enable_operating_limits=ee.enum.enable.no  operating_limit_action=ee.enum.passive.reportOpLim.warn  power_rating=1 W  max_working_voltage=100 V  noise_mode=ee.enum.sources.noise.Disabled  Tdevice=25 degC  sample_time=1e-3 s  repeatability=ee.enum.ic.repeatability.notRepeatable  user_seed=0  auto_seed=2555059182  fault_action=simscape.enum.assert.action.none  t_fault=1 s  power_derating_T1=70 degC  power_derating_T2=155 degC  operating_temperature_range_vec=[-50, 150] degC  alpha=3.93e-3 1/K  Tmeas=25 degC  thermal_mass=100 J/K  temperature_specify=off  temperature_priority=High  temperature=298.15 K  temperature_nominal_specify=off  temperature_nominal_value=1  temperature_nominal_unit=K
  Simscape : Subsystem
      mask Display: disp('V')
  Voltage Source : Subsystem
  dplmodel : Subsystem
  gnd : fl_lib/Electrical/Electrical Elements/Electrical Reference
  a : PMIOPort  Side=Left
  Zvi_out : Outport  VectorParamsAs1DForOutWhenUnconnected=off
  Vnode : Outport  Port=2  VectorParamsAs1DForOutWhenUnconnected=off
  wires:
  [I_A_1] -> Voltage Source/1(I)
  Simscape/1(Out) -> [V_A_1]
  dplmodel/2(hist_out) -> [ho]
  [hi] -> dplmodel/2(hist_in)
  Zvi_in/1 -> [hi]
  [V_A_1] -> dplmodel/1(v), Vnode/1
  dplmodel/1(i) -> [I_A_1]
  [ho] -> Zvi_out/1
  connections:
  Electrical Reference1/LConn1 -- Voltage Source/RConn2
  Resistor1/LConn1 -- gnd/LConn1
  Resistor1/RConn1 -- Voltage Source/RConn1 -- Simscape/LConn1 -- a/RConn1

== system simetranss/Lines/mate_1ph_piline ==
  Capacitor : ee_lib/Passive/Capacitor  cap_option=ee.enum.passive.capacitor.capOption.const  c=C11/2*len F  Cvec=[1e-05, 1e-06] F  Vvec=[0, 10] V  CV_table_symmetry=ee.enum.passive.capacitor.tableSymmetry.yes  f_vec=[1, 10] kHz  DFext_vec=[.8, 1.2]  enable_C_tol=ee.enum.toleranceApplication.none  averaging_period=0 s  C_tol=5  tol_distribution=ee.enum.toleranceDistribution.uniform  nSigma=4  r=0 Ohm  g=0 1/Ohm  enable_operating_limits=ee.enum.enable.no  operating_limit_action=ee.enum.passive.reportOpLim.warn  max_working_voltage_range=[-25, 25] V  power_rating=1 W  maxTemperature=85 degC  thermalEnable=false  thermalMass=1 J/K  fault_action=simscape.enum.assert.action.none  t_fault=1 s  i_specify=off  i_priority=None  i=0 A  i_nominal_specify=off  i_nominal_value=1  i_nominal_unit=A  v_specify=off  v_priority=None  v=0 V  v_nominal_specify=off  v_nominal_value=1  v_nominal_unit=V  vc_specify=off  vc_priority=High  vc=0 V  vc_nominal_specify=off  vc_nominal_value=1  vc_nominal_unit=V  T_specify=off  T_priority=None  T=298.15 K  T_nominal_specify=off  T_nominal_value=1  T_nominal_unit=K
  Capacitor1 : ee_lib/Passive/Capacitor  cap_option=ee.enum.passive.capacitor.capOption.const  c=C11/2*len F  Cvec=[1e-05, 1e-06] F  Vvec=[0, 10] V  CV_table_symmetry=ee.enum.passive.capacitor.tableSymmetry.yes  f_vec=[1, 10] kHz  DFext_vec=[.8, 1.2]  enable_C_tol=ee.enum.toleranceApplication.none  averaging_period=0 s  C_tol=5  tol_distribution=ee.enum.toleranceDistribution.uniform  nSigma=4  r=0 Ohm  g=0 1/Ohm  enable_operating_limits=ee.enum.enable.no  operating_limit_action=ee.enum.passive.reportOpLim.warn  max_working_voltage_range=[-25, 25] V  power_rating=1 W  maxTemperature=85 degC  thermalEnable=false  thermalMass=1 J/K  fault_action=simscape.enum.assert.action.none  t_fault=1 s  i_specify=off  i_priority=None  i=0 A  i_nominal_specify=off  i_nominal_value=1  i_nominal_unit=A  v_specify=off  v_priority=None  v=0 V  v_nominal_specify=off  v_nominal_value=1  v_nominal_unit=V  vc_specify=off  vc_priority=High  vc=0 V  vc_nominal_specify=off  vc_nominal_value=1  vc_nominal_unit=V  T_specify=off  T_priority=None  T=298.15 K  T_nominal_specify=off  T_nominal_value=1  T_nominal_unit=K
  Electrical Reference : fl_lib/Electrical/Electrical Elements/Electrical Reference
  Electrical Reference1 : fl_lib/Electrical/Electrical Elements/Electrical Reference
  Inductor : ee_lib/Passive/Inductor  l=LL*len H  enable_L_tol=ee.enum.toleranceApplication.none  L_tol=20  tol_distribution=ee.enum.toleranceDistribution.uniform  nSigma=4  r=RR*len Ohm  g=1e-9 1/Ohm  enable_operating_limits=ee.enum.enable.no  operating_limit_action=ee.enum.passive.reportOpLim.warn  max_working_current=1 A  power_rating=1 W  fault_action=simscape.enum.assert.action.none  t_fault=1 s  i_L_specify=off  i_L_priority=High  i_L=0 A  i_L_nominal_specify=off  i_L_nominal_value=1  i_L_nominal_unit=A
  a : PMIOPort  Tag=PMCPort  Side=Left
  "a " : PMIOPort  Tag=PMCPort  Port=2  Side=Right
  connections:
  Electrical Reference1/LConn1 -- Capacitor1/RConn1
  Capacitor/RConn1 -- Electrical Reference/LConn1
  Capacitor1/LConn1 -- "a "/RConn1 -- Inductor/RConn1
  a/RConn1 -- Capacitor/LConn1 -- Inductor/LConn1

== system simetranss/Lines/mate_2ph_piline ==
  Capacitor : ee_lib/Passive/Capacitor  cap_option=ee.enum.passive.capacitor.capOption.const  c=C12/2*len F  Cvec=[1e-05, 1e-06] F  Vvec=[0, 10] V  CV_table_symmetry=ee.enum.passive.capacitor.tableSymmetry.yes  f_vec=[1, 10] kHz  DFext_vec=[.8, 1.2]  enable_C_tol=ee.enum.toleranceApplication.none  averaging_period=0 s  C_tol=5  tol_distribution=ee.enum.toleranceDistribution.uniform  nSigma=4  r=0 Ohm  g=0 1/Ohm  enable_operating_limits=ee.enum.enable.no  operating_limit_action=ee.enum.passive.reportOpLim.warn  max_working_voltage_range=[-25, 25] V  power_rating=1 W  maxTemperature=85 degC  thermalEnable=false  thermalMass=1 J/K  fault_action=simscape.enum.assert.action.none  t_fault=1 s  i_specify=off  i_priority=None  i=0 A  i_nominal_specify=off  i_nominal_value=1  i_nominal_unit=A  v_specify=off  v_priority=None  v=0 V  v_nominal_specify=off  v_nominal_value=1  v_nominal_unit=V  vc_specify=off  vc_priority=High  vc=0 V  vc_nominal_specify=off  vc_nominal_value=1  vc_nominal_unit=V  T_specify=off  T_priority=None  T=298.15 K  T_nominal_specify=off  T_nominal_value=1  T_nominal_unit=K
  Capacitor1 : ee_lib/Passive/Capacitor  cap_option=ee.enum.passive.capacitor.capOption.const  c=C12/2*len F  Cvec=[1e-05, 1e-06] F  Vvec=[0, 10] V  CV_table_symmetry=ee.enum.passive.capacitor.tableSymmetry.yes  f_vec=[1, 10] kHz  DFext_vec=[.8, 1.2]  enable_C_tol=ee.enum.toleranceApplication.none  averaging_period=0 s  C_tol=5  tol_distribution=ee.enum.toleranceDistribution.uniform  nSigma=4  r=0 Ohm  g=0 1/Ohm  enable_operating_limits=ee.enum.enable.no  operating_limit_action=ee.enum.passive.reportOpLim.warn  max_working_voltage_range=[-25, 25] V  power_rating=1 W  maxTemperature=85 degC  thermalEnable=false  thermalMass=1 J/K  fault_action=simscape.enum.assert.action.none  t_fault=1 s  i_specify=off  i_priority=None  i=0 A  i_nominal_specify=off  i_nominal_value=1  i_nominal_unit=A  v_specify=off  v_priority=None  v=0 V  v_nominal_specify=off  v_nominal_value=1  v_nominal_unit=V  vc_specify=off  vc_priority=High  vc=0 V  vc_nominal_specify=off  vc_nominal_value=1  vc_nominal_unit=V  T_specify=off  T_priority=None  T=298.15 K  T_nominal_specify=off  T_nominal_value=1  T_nominal_unit=K
  Capacitor2 : ee_lib/Passive/Capacitor  cap_option=ee.enum.passive.capacitor.capOption.const  c=C11/2*len F  Cvec=[1e-05, 1e-06] F  Vvec=[0, 10] V  CV_table_symmetry=ee.enum.passive.capacitor.tableSymmetry.yes  f_vec=[1, 10] kHz  DFext_vec=[.8, 1.2]  enable_C_tol=ee.enum.toleranceApplication.none  averaging_period=0 s  C_tol=5  tol_distribution=ee.enum.toleranceDistribution.uniform  nSigma=4  r=0 Ohm  g=0 1/Ohm  enable_operating_limits=ee.enum.enable.no  operating_limit_action=ee.enum.passive.reportOpLim.warn  max_working_voltage_range=[-25, 25] V  power_rating=1 W  maxTemperature=85 degC  thermalEnable=false  thermalMass=1 J/K  fault_action=simscape.enum.assert.action.none  t_fault=1 s  i_specify=off  i_priority=None  i=0 A  i_nominal_specify=off  i_nominal_value=1  i_nominal_unit=A  v_specify=off  v_priority=None  v=0 V  v_nominal_specify=off  v_nominal_value=1  v_nominal_unit=V  vc_specify=off  vc_priority=High  vc=0 V  vc_nominal_specify=off  vc_nominal_value=1  vc_nominal_unit=V  T_specify=off  T_priority=None  T=298.15 K  T_nominal_specify=off  T_nominal_value=1  T_nominal_unit=K
  Capacitor3 : ee_lib/Passive/Capacitor  cap_option=ee.enum.passive.capacitor.capOption.const  c=C22/2*len F  Cvec=[1e-05, 1e-06] F  Vvec=[0, 10] V  CV_table_symmetry=ee.enum.passive.capacitor.tableSymmetry.yes  f_vec=[1, 10] kHz  DFext_vec=[.8, 1.2]  enable_C_tol=ee.enum.toleranceApplication.none  averaging_period=0 s  C_tol=5  tol_distribution=ee.enum.toleranceDistribution.uniform  nSigma=4  r=0 Ohm  g=0 1/Ohm  enable_operating_limits=ee.enum.enable.no  operating_limit_action=ee.enum.passive.reportOpLim.warn  max_working_voltage_range=[-25, 25] V  power_rating=1 W  maxTemperature=85 degC  thermalEnable=false  thermalMass=1 J/K  fault_action=simscape.enum.assert.action.none  t_fault=1 s  i_specify=off  i_priority=None  i=0 A  i_nominal_specify=off  i_nominal_value=1  i_nominal_unit=A  v_specify=off  v_priority=None  v=0 V  v_nominal_specify=off  v_nominal_value=1  v_nominal_unit=V  vc_specify=off  vc_priority=High  vc=0 V  vc_nominal_specify=off  vc_nominal_value=1  vc_nominal_unit=V  T_specify=off  T_priority=None  T=298.15 K  T_nominal_specify=off  T_nominal_value=1  T_nominal_unit=K
  Capacitor4 : ee_lib/Passive/Capacitor  cap_option=ee.enum.passive.capacitor.capOption.const  c=C22/2*len F  Cvec=[1e-05, 1e-06] F  Vvec=[0, 10] V  CV_table_symmetry=ee.enum.passive.capacitor.tableSymmetry.yes  f_vec=[1, 10] kHz  DFext_vec=[.8, 1.2]  enable_C_tol=ee.enum.toleranceApplication.none  averaging_period=0 s  C_tol=5  tol_distribution=ee.enum.toleranceDistribution.uniform  nSigma=4  r=0 Ohm  g=0 1/Ohm  enable_operating_limits=ee.enum.enable.no  operating_limit_action=ee.enum.passive.reportOpLim.warn  max_working_voltage_range=[-25, 25] V  power_rating=1 W  maxTemperature=85 degC  thermalEnable=false  thermalMass=1 J/K  fault_action=simscape.enum.assert.action.none  t_fault=1 s  i_specify=off  i_priority=None  i=0 A  i_nominal_specify=off  i_nominal_value=1  i_nominal_unit=A  v_specify=off  v_priority=None  v=0 V  v_nominal_specify=off  v_nominal_value=1  v_nominal_unit=V  vc_specify=off  vc_priority=High  vc=0 V  vc_nominal_specify=off  vc_nominal_value=1  vc_nominal_unit=V  T_specify=off  T_priority=None  T=298.15 K  T_nominal_specify=off  T_nominal_value=1  T_nominal_unit=K
  Capacitor5 : ee_lib/Passive/Capacitor  cap_option=ee.enum.passive.capacitor.capOption.const  c=C11/2*len F  Cvec=[1e-05, 1e-06] F  Vvec=[0, 10] V  CV_table_symmetry=ee.enum.passive.capacitor.tableSymmetry.yes  f_vec=[1, 10] kHz  DFext_vec=[.8, 1.2]  enable_C_tol=ee.enum.toleranceApplication.none  averaging_period=0 s  C_tol=5  tol_distribution=ee.enum.toleranceDistribution.uniform  nSigma=4  r=0 Ohm  g=0 1/Ohm  enable_operating_limits=ee.enum.enable.no  operating_limit_action=ee.enum.passive.reportOpLim.warn  max_working_voltage_range=[-25, 25] V  power_rating=1 W  maxTemperature=85 degC  thermalEnable=false  thermalMass=1 J/K  fault_action=simscape.enum.assert.action.none  t_fault=1 s  i_specify=off  i_priority=None  i=0 A  i_nominal_specify=off  i_nominal_value=1  i_nominal_unit=A  v_specify=off  v_priority=None  v=0 V  v_nominal_specify=off  v_nominal_value=1  v_nominal_unit=V  vc_specify=off  vc_priority=High  vc=0 V  vc_nominal_specify=off  vc_nominal_value=1  vc_nominal_unit=V  T_specify=off  T_priority=None  T=298.15 K  T_nominal_specify=off  T_nominal_value=1  T_nominal_unit=K
  Coupled Lines (Pair) : ee_lib/Passive/Lines/Coupled Lines (Pair)  prm=2  L1=LL(1,1)*len H  L2=LL(2,2)*len H  L=1e-3 H  Lm=LL(1,2)*len H  R1=RR(1,1)*len Ohm  R2=RR(2,2)*len Ohm  R=0.001 Ohm  Rm=RR(1,2)*len Ohm  G1=1e-9 1/Ohm  G2=1e-9 1/Ohm  G=1e-9 1/Ohm  i_L1_specify=off  i_L1_priority=High  i_L1=0 A  i_L1_nominal_specify=off  i_L1_nominal_value=1  i_L1_nominal_unit=A  i_L2_specify=off  i_L2_priority=High  i_L2=0 A  i_L2_nominal_specify=off  i_L2_nominal_value=1  i_L2_nominal_unit=A
      settings: InternalSimscapePortConfiguration="{\"Bottom\":[],\"Left\":[{\"id\":\"p1\",\"label\":\"1+\",\"type\":\"foundation.electrical.electrical\"},{\"id\":\"p2\",\"label\":\"2+\",\"type\":\"foundation.electrical.electrical\"}],\"Right\":[{\"id\":\"n1\",\"label\":\"1-\",\"type\":\"foundation.electrical.electrical\"},{\"id\":\"n2\",\"label\":\"2-\",\"type\":\"foundation.electrical.electrical\"}],\"Top\":[]}"
  Electrical Reference{,1..3} (4 alike) : fl_lib/Electrical/Electrical Elements/Electrical Reference
  a : PMIOPort  Tag=PMCPort  Side=Left
  b : PMIOPort  Tag=PMCPort  Port=2  Side=Left
  "a " : PMIOPort  Tag=PMCPort  Port=3  Side=Right
  "b " : PMIOPort  Tag=PMCPort  Port=4  Side=Right
  connections:
  Electrical Reference/LConn1 -- Capacitor2/RConn1
  Electrical Reference1/LConn1 -- Capacitor3/RConn1
  Electrical Reference2/LConn1 -- Capacitor4/RConn1
  Electrical Reference3/LConn1 -- Capacitor5/RConn1
  a/RConn1 -- Capacitor/LConn1 -- Capacitor2/LConn1 -- Coupled Lines (Pair)/LConn1
  b/RConn1 -- Capacitor/RConn1 -- Coupled Lines (Pair)/LConn2 -- Capacitor3/LConn1
  Capacitor1/LConn1 -- "a "/RConn1 -- Coupled Lines (Pair)/RConn1 -- Capacitor5/LConn1
  Capacitor1/RConn1 -- "b "/RConn1 -- Coupled Lines (Pair)/RConn2 -- Capacitor4/LConn1
